simulink model "FOC_PMSM_FVSensorNew"  (R2019b)
settings: Solver=ode45  StartTime=0  StopTime=1  FixedStep=1/fs/4  MaxStep=1/fs/2  RelTol=1e-7  EnableMultiTasking=on
InitFcn:
  | Motor_parameters_Lsrpm7fw
values from neighbouring files (symbols this model uses):
  fs = 20e3    (= 20000)    [Motor_parameters_Lsrpm7fw.m]
  Iphmax = I_rated*sqrt(2)*3    [Motor_parameters_Lsrpm7fw.m]
  J = 1*1e-3    (= 0.001)    [Motor_parameters_Lsrpm7fw.m]
  Ki1 = 2    [Motor_parameters_Lsrpm7fw.m]
  Ki2 = 6000    [Motor_parameters_Lsrpm7fw.m]
  Ki_pll = Bw^2*(1.1-0.334*zeta)^2*1/(2*k1)    (= 1705731.55439)    [Motor_parameters_Lsrpm7fw.m]
  Kp1 = 0.005    [Motor_parameters_Lsrpm7fw.m]
  Kp2 = 6    [Motor_parameters_Lsrpm7fw.m]
  Kp_pll = Bw*(2.2*zeta-0.668*zeta^2)*1/(2*k1)    (= 27920.01984)    [Motor_parameters_Lsrpm7fw.m]
  Ld = 10e-3    (= 0.01)    [Motor_parameters_Lsrpm7fw.m]
  Lndd_ini = Lndmpm    (= 0.412)    [Motor_parameters_Lsrpm7fw.m]
  Lndmpm = 0.412    [Motor_parameters_Lsrpm7fw.m]
  Lq = 12.8e-3    (= 0.0128)    [Motor_parameters_Lsrpm7fw.m]
  Npp = 8/2    (= 4)    [Motor_parameters_Lsrpm7fw.m]
  Omegae_ini = 0    [Motor_parameters_Lsrpm7fw.m]
  Rs = 0.78    [Motor_parameters_Lsrpm7fw.m]
  Tl_const = Trat/nrat^2    (= 1.24081632653e-05)    [Motor_parameters_Lsrpm7fw.m]
  Trat = 38    [Motor_parameters_Lsrpm7fw.m]
  Vm = 70    [Motor_parameters_Lsrpm7fw.m]
  Vph = Vs*sqrt(2)    [Motor_parameters_Lsrpm7fw.m]
undefined symbols (not defined in the file or in its folder): DiscIntNeverNeededParam, plecs, sigbuilder_block
libraries: simulink x1
(part 1 of 2)
settings Model: Creator=klu  LastModifiedBy=Kristina
settings SolverCC: AlgebraicLoopSolver=LineSearch
settings DataIOCC: LimitDataPoints=on  SaveFormat=Array  SignalLoggingSaveFormat=ModelDataLogs  ReturnWorkspaceOutputs=off
settings OptimizationCC: BooleanDataType=off  ExpressionDepthLimit=2147483647  InitFltsAndDblsToZero=on  LifeSpan=inf
settings DebuggingCC: AlgebraicLoopMsg=none  SaveWithParameterizedLinksMsg=none  UnderspecifiedInitializationDetection=Classic  MergeDetectMultiDrivingBlocksExec=none  SignalResolutionControl=TryResolveAllWithWarning  MultiTaskDSMMsg=warning  MultiTaskCondExecSysMsg=none  FcnCallInpInsideContextMsg=warning  StateNameClashWarn=warning  SFUnexpectedBacktrackingDiag=warning  SFNoUnconditionalDefaultTransitionDiag=warning  SFExecutionAtInitializationDiag=none  ArithmeticOperatorsInVariantConditions=warning
settings HardwareCC: ProdBitPerPointer=32  ProdBitPerSizeT=32  ProdBitPerPtrDiffT=32  ProdLargestAtomicFloat=None  ProdIntDivRoundTo=Undefined  ProdEndianess=Unspecified  ProdWordSize=32  ProdHWDeviceType=32-bit Generic
settings ModelReferenceCC: PropagateSignalLabelsOutOfModel=off
settings SFSimCC: SimUseLocalCustomCode=off  CustomCodeUndefinedFunction=UseInterfaceOnly
settings RTWCC: RTWUseLocalCustomCode=off
settings CodeAppCC: StateflowObjectComments=on
settings GRTTargetCC: TargetFcnLib=ansi_tfl_tmw.mat  TargetLangStandard=C89/C90 (ANSI)  GeneratePreprocessorConditionals=Disable all  CombineOutputUpdateFcns=off  GRTInterface=on
settings ConfigComp: CovMetricSettings=dw  CovHtmlReporting=on  CovSaveCumulativeToWorkspaceVar=on  CovSaveSingleToWorkspaceVar=on  CovExternalEMLEnable=off  CovSFcnEnable=off

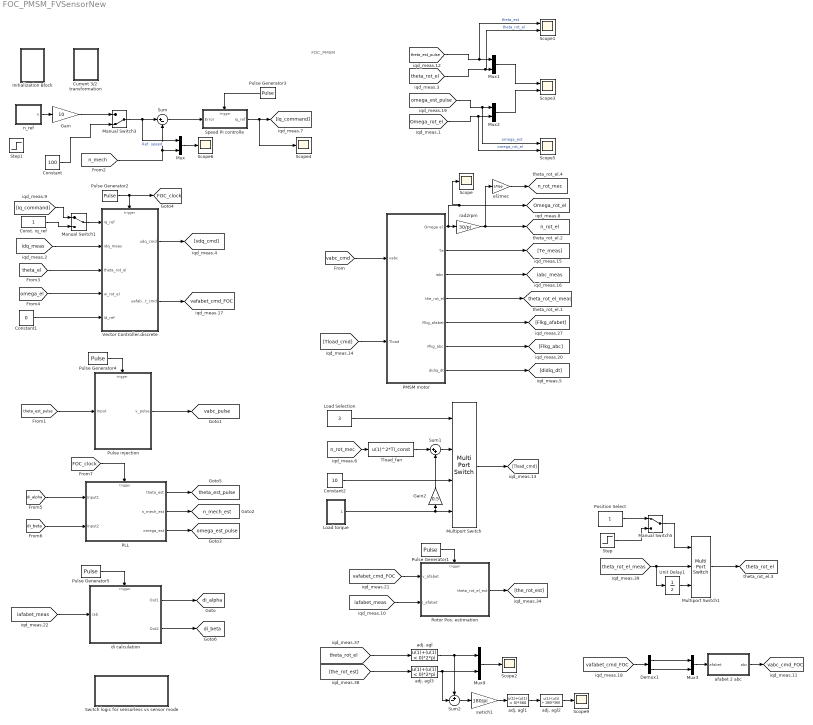
== system FOC_PMSM_FVSensorNew ==
  note: FOC_PMSM
  Const. iq_ref : Constant
  Constant : Constant  Value=100
  Constant1 : Constant  Value=0
  Constant2 : Constant  Value=10
  Current 3/2 transformation : Subsystem
      mask Display:
      | plot([0.1000    0.1357    0.1714    0.2071    0.2429    0.2786    0.3143    0.3500    0.3857    0.4214 0.4571    0.4929    0.5286    0.5643    0.6000]-0.05,0.4+0.6*[0.5000    0.5868    0.6564    0.6950    0.6950    0.6564    0.5868    0.5000    0.4132    0.3436 0.3050    0.3050    0.3436    0.4132    0.5000])
      | 
      | plot([0.1,0.9],[0.1,0.9])
      | 
      | plot([0.5,0.9],0.3*[1 1])
  Demux1 : Demux  Outputs=2
  Gain : Gain  Gain=10
  Gain2 : Gain  Gain=0.5
  Initialization Block : Subsystem  mask{init_in=Motor_parameters_Lsrpm7fw}
      mask prompts: init_in "Enter Initialization Script:"
      mask init:
      | aaa =3;
      mask Callback init_in:
      | init_script=get_param(gcb,'MaskValueString');
      | %eval(init_script);
      | %set_param(gcs,'PreLoadFcn',init_script)
      | set_param(gcs,'InitFcn',init_script)
      | 
      | % Change the parameters here;
      | Ld               = Ld;
      | Lq               = Ld;
  Load Selection : Constant  Value=3
  Load torque : Subsystem
  Manual Switch1 : ManualSwitch
  Manual Switch3 : ManualSwitch  CurrentSetting=0
  Manual Switch5 : ManualSwitch
  Multiport Switch : MultiPortSwitch
  Multiport Switch1 : MultiPortSwitch  Inputs=2
  Mux{,1..3,9} (5 alike) : Mux  Inputs=2
  PLL : Subsystem  TreatAsAtomicUnit=on
  PMSM motor : Subsystem
  Position Select : Constant
  Pulse Generator1 : DiscretePulseGenerator  PulseType=Time based  Period=1/fs  PulseWidth=50  PhaseDelay=1/fs/4*0
  Pulse Generator2 : DiscretePulseGenerator  PulseType=Time based  Period=1/fs  PulseWidth=50
  Pulse Generator3 : DiscretePulseGenerator  PulseType=Time based  Period=1/fs  PulseWidth=50
  Pulse Generator4 : DiscretePulseGenerator  PulseType=Time based  Period=1/fs  PulseWidth=50  PhaseDelay=(1/fs)*0.5
  Pulse Generator5 : DiscretePulseGenerator  PulseType=Time based  Period=1/(fs*2)  PulseWidth=50
  Pulse injection : Subsystem  TreatAsAtomicUnit=on
  Rotor Pos. estimation : Subsystem
  Scope{,2,4,6,9} (5 alike) : Scope
  Scope1 : Scope  NumInputPorts=2
  Scope3 : Scope  NumInputPorts=2
  Scope5 : Scope  NumInputPorts=2
  Speed PI controlle : Subsystem
  Step : Step  Time=0  Before=1  After=2  SampleTime=0
  Step1 : Step  Time=0.2  Before=100  After=100  SampleTime=0
  Sum : Sum  Inputs=|+-
  Sum1 : Sum  Inputs=|++
  Sum2 : Sum  Inputs=+-|
  Switch logic for sensorless vs sensor mode : Subsystem
  Tload_fan : Fcn  Expr=u(1)^2*Tl_const
  Unit Delay1 : UnitDelay  SampleTime=(1/fs)*4  HasFrameUpgradeWarning=on
  Vector Controller.discrete : Subsystem
  adj. agl : Fcn  Expr=u(1)+(u(1) < 0)*2*pi
  adj. agl1 : Fcn  Expr=u(1)+(u(1) < 0)*360
  adj. agl2 : Fcn  Expr=u(1)-(u(1) > 180)*360
  adj. agl3 : Fcn  Expr=u(1)+(u(1) < 0)*2*pi
  afabet 2 abc : Subsystem
  di calculation : Subsystem  TreatAsAtomicUnit=on
  el2mec : Gain  Gain=1/Npp
  n_ref : Subsystem  Tag=STV Subsys  LoadFcn=sigbuilder_block('load');  StartFcn=sigbuilder_block('start');  StopFcn=sigbuilder_block('stop');  ClipboardFcn=sigbuilder_block('clipboard');  mask(Sigbuilder block){tuvar=[0:10]}
      mask help: Sigbuilder GUI
      mask init:
      | if ~strcmp(get_param(bdroot(gcbh),'SimulationStatus'),'stopped') tuvar = sigbuilder_block('maskInit'); end
      settings: CopyFcn=sigbuilder_block('copy');  DeleteFcn=sigbuilder_block('delete');  ModelCloseFcn=sigbuilder_block('modelClose');  PreSaveFcn=sigbuilder_block('preSave');  PauseFcn=sigbuilder_block('pause')  ContinueFcn=sigbuilder_block('continue')  NameChangeFcn=sigbuilder_block('namechange');  OpenFcn=sigbuilder_block('open',[72.75 116.25 550.5 363.75 ]);  CloseFcn=sigbuilder_block('close');
      mask Display: plot(0, 0, 100, 100,[2, 2, 32, 32, 2], [68, 8, 8, 68, 68],[32, 2], [38, 38], [32, 19, 2],[53, 60, 44], [32, 17, 17, 2],[16, 16, 31, 31]);txt = getActiveGroup(gcbh);text(2, 100, txt,'verticalAlignment', 'top');
  rad2rpm : Gain  Gain=30/pi
  swtich1 : Gain  Gain=180/pi
  tag scope: FOC_clock=global, Omega_rot_el=global, di_alpha=global, di_beta=global, iabc_meas=global, n_mech_est=global, n_rot_el=global, n_rot_mec=global, omega_est_pulse=global, theta_est_pulse=global, theta_rot_el=global, theta_rot_el_meas=global, vabc_cmd_FOC=global, vabc_pulse=global, vafabet_cmd_FOC=global
  wires:
  Manual Switch1/1 -> Vector Controller.discrete/1(iq_ref)
  Const. iq_ref/1 -> Manual Switch1/2
  Sum/1 -> Speed PI controlle/1(Error)
  [idq_meas] -> Vector Controller.discrete/2(idq_meas)
  Vector Controller.discrete/1(udq_cmd) -> [vdq_cmd]
  Vector Controller.discrete/2(uafabet_cmd) -> [vafabet_cmd_FOC]
  Constant2/1 -> Multiport Switch/3
  Load torque/1(T_load) -> Multiport Switch/4, Gain2/1
  Multiport Switch/1 -> [Tload_cmd]
  [n_rot_mec] -> Tload_fan/1
  Load Selection/1 -> Multiport Switch/1
  [theta_rot_el_meas] -> Unit Delay1/1, Multiport Switch1/2
  Multiport Switch1/1 -> [theta_rot_el]
  Position Select/1 -> Manual Switch5/1
  Step/1 -> Manual Switch5/2
  Manual Switch5/1 -> Multiport Switch1/1
  n_ref/1(n) -> Gain/1
  Gain/1 -> Manual Switch3/1
  Sum1/1 -> Multiport Switch/2
  Tload_fan/1 -> Sum1/1
  [theta_el] -> Vector Controller.discrete/3(theta_rot_el)
  Constant1/1 -> Vector Controller.discrete/5(Id_ref)
  Gain2/1 -> Sum1/2
  Unit Delay1/1 -> Multiport Switch1/3
  [omega_el] -> Vector Controller.discrete/4(w_rot_el)
  PMSM motor/2(Te) -> [Te_meas]
  PMSM motor/1(Omega el.) -> Scope/1, [Omega_rot_el], rad2rpm/1
  rad2rpm/1 -> [n_rot_el], el2mec/1
  PMSM motor/5(Flkg_afabet) -> [Flkg_afabet]
  PMSM motor/6(Flkg_abc) -> [Flkg_abc]
  [Tload_cmd] -> PMSM motor/2(Tload)
  PMSM motor/3(iabc) -> [iabc_meas]
  PMSM motor/7(didiq_dt) -> [didiq_dt]
  Demux1/2 -> Mux3/2
  Demux1/1 -> Mux3/1
  [vafabet_cmd_FOC] -> Demux1/1
  afabet 2 abc/1(abc) -> [vabc_cmd_FOC]
  Mux3/1 -> afabet 2 abc/1(afabet)
  Speed PI controlle/1(iq_ref) -> Scope4/1, [Iq_command]
  [Iq_command] -> Manual Switch1/1
  adj. agl1/1 -> adj. agl2/1
  [the_rot_est] -> adj. agl3/1
  adj. agl2/1 -> Scope9/1
  [iafabet_meas] -> Rotor Pos. estimation/2(i_afabet)
  swtich1/1 -> adj. agl1/1
  Sum2/1 -> swtich1/1
  [vafabet_cmd_FOC] -> Rotor Pos. estimation/1(v_afabet)
  Rotor Pos. estimation/1(theta_rot_el_est) -> [the_rot_est]
  adj. agl/1 -> Mux9/1, Sum2/1
  [theta_rot_el] -> adj. agl/1
  Pulse Generator1/1 -> Rotor Pos. estimation/Trigger
  adj. agl3/1 -> Mux9/2, Sum2/2
  el2mec/1 -> [n_rot_mec]
  Pulse Generator3/1 -> Speed PI controlle/Trigger
  Mux9/1 -> Scope2/1
  Pulse Generator4/1 -> Pulse injection/Trigger
  Pulse Generator2/1 -> [FOC_clock], Vector Controller.discrete/Trigger
  [iafabet_meas] -> di calculation/1(iab)
  Pulse injection/1(v_pulse) -> [vabc_pulse]
  Manual Switch3/1 -> Mux/1, Sum/1  "Ref. speed"
  Mux/1 -> Scope6/1
  [n_mech] -> Mux/2, Sum/2
  [vabc_cmd] -> PMSM motor/1(vabc)
  Pulse Generator5/1 -> di calculation/Trigger
  PMSM motor/4(the_rot_el) -> [theta_rot_el_meas]
  PLL/1(theta_est) -> [theta_est_pulse]
  PLL/2(n_mech_est) -> [n_mech_est]
  PLL/3(omega_est) -> [omega_est_pulse]
  [theta_est_pulse] -> Pulse injection/1(Input)
  di calculation/1(Out1) -> [di_alpha]
  di calculation/2(Out2) -> [di_beta]
  [di_alpha] -> PLL/1(Input1)
  [di_beta] -> PLL/2(Input2)
  [FOC_clock] -> PLL/Trigger
  [theta_est_pulse] -> Scope1/1, Mux1/1  "theta_est"
  [theta_rot_el] -> Scope1/2, Mux1/2  "theta_rot_el"
  [omega_est_pulse] -> Scope5/1, Mux2/1  "omega_est"
  [Omega_rot_el] -> Scope5/2, Mux2/2  "omega_rot_el"
  Mux1/1 -> Scope3/1
  Mux2/1 -> Scope3/2
  Constant/1 -> Manual Switch3/2

== system FOC_PMSM_FVSensorNew/Current 3//2 transformation ==
  Delay : Delay  DelayLength=1
  Detect peak : Subsystem
  Display : Display
  Display1 : Display
  Manual Switch7 : ManualSwitch  CurrentSetting=0
  Scope14 : Scope
  Scope6 : Scope
  abc 2 dq : Subsystem
  dq 2 afa beta : Subsystem
  tag scope: iafabet_meas=global, idq_meas=global
  wires:
  abc 2 dq/1(dq) -> [idq_meas], Scope6/1, dq 2 afa beta/1(dq)
  dq 2 afa beta/1(afa beta) -> [iafabet_meas], Scope14/1
  Manual Switch7/1 -> abc 2 dq/1(abc), Detect peak/1(iabc)
  Detect peak/1(Peak) -> Display/1
  [iabc_meas] -> Manual Switch7/1, Manual Switch7/2
  [theta_el] -> Delay/1, Display1/1
  Delay/1 -> abc 2 dq/2(theta), dq 2 afa beta/2(theta)

== system FOC_PMSM_FVSensorNew/Initialization Block ==

== system FOC_PMSM_FVSensorNew/Load torque ==
  Add : Sum  Inputs=+++
  Scope2 : Scope
  Step Load torque 1 : Step  Time=2  After=Trat  SampleTime=0
  Step Load torque2 : Step  Time=4  After=-Trat/2  SampleTime=0
  Tload : Constant  Value=0
  T_load : Outport  VectorParamsAs1DForOutWhenUnconnected=off
  wires:
  Tload/1 -> Add/1
  Step Load torque 1/1 -> Add/2
  Step Load torque2/1 -> Add/3
  Add/1 -> T_load/1, Scope2/1

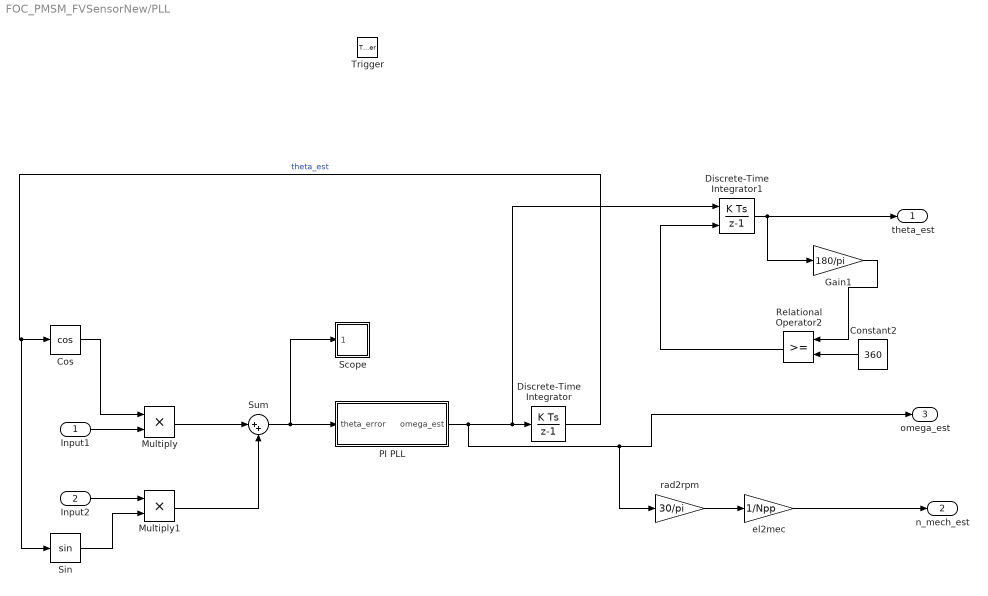
== system FOC_PMSM_FVSensorNew/PLL ==
  Input1 : Inport
  Input2 : Inport  Port=2
  Trigger : TriggerPort  VariantControl=Variant
  Constant2 : Constant  Value=360
  Cos : Trigonometry  Operator=cos
  Discrete-Time Integrator : DiscreteIntegrator  SampleTime=-1  ICPrevOutput=DiscIntNeverNeededParam  ICPrevScaledInput=DiscIntNeverNeededParam
  Discrete-Time Integrator1 : DiscreteIntegrator  ExternalReset=rising  SampleTime=-1  ICPrevOutput=DiscIntNeverNeededParam  ICPrevScaledInput=DiscIntNeverNeededParam
  Gain1 : Gain  Gain=180/pi
  Multiply : Product
  Multiply1 : Product
  PI PLL : Subsystem
  Relational Operator2 : RelationalOperator  OutDataTypeStr=boolean  RndMeth=Nearest
  Scope : Subsystem  LoadFcn=plecs('sl', 300);  InitFcn=plecs('sl', 314);  StartFcn=plecs('sl', 308);  StopFcn=plecs('sl', 309);  mask{Settings=<binary blob, 232 chars, not shown>}
      mask init:
      | plecs('sl', 315);
      settings: CopyFcn=plecs('sl', 303);  DeleteFcn=plecs('sl', 305);  UndoDeleteFcn=plecs('sl', 306);  PreSaveFcn=plecs('sl', 311);  NameChangeFcn=plecs('sl', 310);  DestroyFcn=plecs('sl', 307);  OpenFcn=plecs('sl', 302);  ErrorFcn=plerrorfcn
      mask Display: plot([0.1 0.9 0.9 0.1 0.1], [0.9 0.9 0.5 0.5 0.9])
  Sin : Trigonometry
  Sum : Sum  Inputs=|++
  el2mec : Gain  Gain=1/Npp
  rad2rpm : Gain  Gain=30/pi
  theta_est : Outport  VectorParamsAs1DForOutWhenUnconnected=off
  n_mech_est : Outport  Port=2  VectorParamsAs1DForOutWhenUnconnected=off
  omega_est : Outport  Port=3  VectorParamsAs1DForOutWhenUnconnected=off
  wires:
  el2mec/1 -> n_mech_est/1
  Sum/1 -> Scope/1(1), PI PLL/1(theta_error)
  Multiply/1 -> Sum/1
  Relational Operator2/1 -> Discrete-Time Integrator1/2
  Input2/1 -> Multiply1/1
  Gain1/1 -> Relational Operator2/1
  Discrete-Time Integrator1/1 -> Gain1/1, theta_est/1
  Cos/1 -> Multiply/1
  Sin/1 -> Multiply1/2
  Input1/1 -> Multiply/2
  rad2rpm/1 -> el2mec/1
  Discrete-Time Integrator/1 -> Sin/1, Cos/1  "theta_est"
  PI PLL/1(omega_est) -> rad2rpm/1, omega_est/1, Discrete-Time Integrator1/1, Discrete-Time Integrator/1
  Constant2/1 -> Relational Operator2/2
  Multiply1/1 -> Sum/2

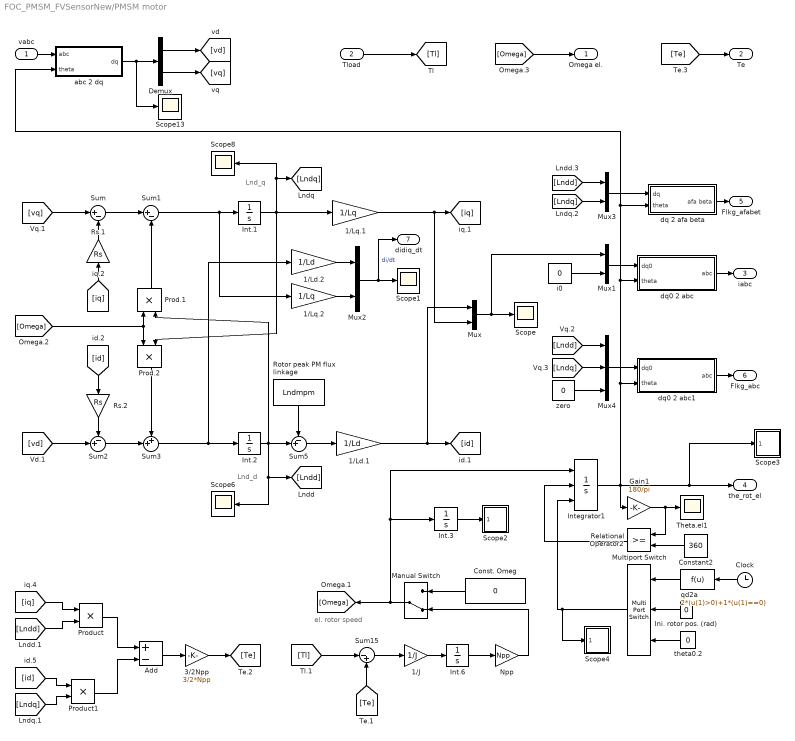
== system FOC_PMSM_FVSensorNew/PMSM motor ==
  note: Lnd_d
  note: Lnd_q
  note: el. rotor speed
  vabc : Inport
  Tload : Inport  Port=2
  1/J : Gain  Gain=1/J
  1/Ld.1 : Gain  Gain=1/Ld
  1/Ld.2 : Gain  Gain=1/Ld
  1/Lq.1 : Gain  Gain=1/Lq
  1/Lq.2 : Gain  Gain=1/Lq
  3/2Npp : Gain  Gain=3/2*Npp
  Add : Sum  Inputs=+-
  Clock : Clock
  Const. Omeg : Constant  Value=0
  Constant2 : Constant  Value=360
  Demux : Demux  Outputs=2
  Gain1 : Gain  Gain=180/pi
  Ini. rotor pos. (rad) : Constant  Value=0
  Int.1 : Integrator
  Int.2 : Integrator  InitialCondition=Lndd_ini
  Int.3 : Integrator  InitialCondition=Omegae_ini/Npp
  Int.6 : Integrator  InitialCondition=Omegae_ini/Npp
  Integrator1 : Integrator  ExternalReset=rising  InitialConditionSource=external  InitialCondition=pi/3
  Manual Switch : ManualSwitch  CurrentSetting=0
  Multiport Switch : MultiPortSwitch  Inputs=2
  Mux{,1..3} (4 alike) : Mux  Inputs=2
  Mux4 : Mux  Inputs=3
  Npp : Gain  Gain=Npp
  Prod.1 : Product  RndMeth=Zero
  Prod.2 : Product  RndMeth=Zero
  Product : Product  RndMeth=Zero
  Product1 : Product  RndMeth=Zero
  Relational Operator2 : RelationalOperator  OutDataTypeStr=boolean  RndMeth=Nearest
  Rotor peak PM flux linkage : Constant  Value=Lndmpm
  Rs.1 : Gain  Gain=Rs
  Rs.2 : Gain  Gain=Rs
  Scope{,1,6,8,13} (5 alike) : Scope
  Scope2 : Subsystem  LoadFcn=plecs('sl', 300);  InitFcn=plecs('sl', 314);  StartFcn=plecs('sl', 308);  StopFcn=plecs('sl', 309);  mask{Settings=<binary blob, 1052 chars, not shown>}
      mask init:
      | plecs('sl', 315);
      settings: CopyFcn=plecs('sl', 303);  DeleteFcn=plecs('sl', 305);  UndoDeleteFcn=plecs('sl', 306);  PreSaveFcn=plecs('sl', 311);  NameChangeFcn=plecs('sl', 310);  DestroyFcn=plecs('sl', 307);  OpenFcn=plecs('sl', 302);  ErrorFcn=plerrorfcn
      mask Display: plot([0.1 0.9 0.9 0.1 0.1], [0.9 0.9 0.5 0.5 0.9])
  Scope3 : Subsystem  LoadFcn=plecs('sl', 300);  InitFcn=plecs('sl', 314);  StartFcn=plecs('sl', 308);  StopFcn=plecs('sl', 309);  mask{Settings=<binary blob, 1052 chars, not shown>}
      mask init:
      | plecs('sl', 315);
      settings: CopyFcn=plecs('sl', 303);  DeleteFcn=plecs('sl', 305);  UndoDeleteFcn=plecs('sl', 306);  PreSaveFcn=plecs('sl', 311);  NameChangeFcn=plecs('sl', 310);  DestroyFcn=plecs('sl', 307);  OpenFcn=plecs('sl', 302);  ErrorFcn=plerrorfcn
      mask Display: plot([0.1 0.9 0.9 0.1 0.1], [0.9 0.9 0.5 0.5 0.9])
  Scope4 : Subsystem  LoadFcn=plecs('sl', 300);  InitFcn=plecs('sl', 314);  StartFcn=plecs('sl', 308);  StopFcn=plecs('sl', 309);  mask{Settings=<binary blob, 1052 chars, not shown>}
      mask init:
      | plecs('sl', 315);
      settings: CopyFcn=plecs('sl', 303);  DeleteFcn=plecs('sl', 305);  UndoDeleteFcn=plecs('sl', 306);  PreSaveFcn=plecs('sl', 311);  NameChangeFcn=plecs('sl', 310);  DestroyFcn=plecs('sl', 307);  OpenFcn=plecs('sl', 302);  ErrorFcn=plerrorfcn
      mask Display: plot([0.1 0.9 0.9 0.1 0.1], [0.9 0.9 0.5 0.5 0.9])
  Sum : Sum  Inputs=|+-
  Sum1 : Sum  Inputs=|+-
  Sum15 : Sum  Inputs=|-+
  Sum2 : Sum  Inputs=-+|
  Sum3 : Sum  Inputs=++|
  Sum5 : Sum  Inputs=-+|
  Theta.el1 : Scope
  abc 2 dq : Subsystem
  dq 2 afa beta : Subsystem
  dq0 2 abc : Subsystem
  dq0 2 abc1 : Subsystem
  i0 : Constant  Value=0
  qd2a : Fcn  Expr=2*(u(1)>0)+1*(u(1)==0)
  theta0.2 : Constant  Value=0
  zero : Constant  Value=0
  Omega el. : Outport  VectorParamsAs1DForOutWhenUnconnected=off
  Te : Outport  Port=2  VectorParamsAs1DForOutWhenUnconnected=off
  iabc : Outport  Port=3  VectorParamsAs1DForOutWhenUnconnected=off
  the_rot_el : Outport  Port=4  VectorParamsAs1DForOutWhenUnconnected=off
  Flkg_afabet : Outport  Port=5  VectorParamsAs1DForOutWhenUnconnected=off
  Flkg_abc : Outport  Port=6  VectorParamsAs1DForOutWhenUnconnected=off
  didiq_dt : Outport  Port=7  VectorParamsAs1DForOutWhenUnconnected=off
  wires:
  3/2Npp/1 -> [Te]
  Add/1 -> 3/2Npp/1
  Sum5/1 -> 1/Ld.1/1
  Rotor peak PM flux linkage/1 -> Sum5/1
  [Omega] -> Omega el./1
  [Te] -> Te/1
  Product1/1 -> Add/2
  Product/1 -> Add/1
  [Lndq] -> Product1/2
  [id] -> Product1/1
  [Te] -> Sum15/2
  Int.6/1 -> Npp/1
  1/J/1 -> Int.6/1
  Sum15/1 -> 1/J/1
  [Tl] -> Sum15/1
  Mux/1 -> Scope/1, Mux1/1
  [Omega] -> Prod.2/1, Prod.1/1
  Sum3/1 -> Int.2/1, 1/Ld.2/1
  Prod.2/1 -> Sum3/1
  Sum2/1 -> Sum3/2
  [id] -> Rs.2/1
  Rs.2/1 -> Sum2/1
  [vd] -> Sum2/2
  1/Ld.1/1 -> [id], Mux/1
  Int.2/1 -> [Lndd], Scope6/1, Sum5/2, Prod.1/2
  [iq] -> Rs.1/1
  1/Lq.1/1 -> [iq], Mux/2
  Prod.1/1 -> Sum1/2
  Sum1/1 -> Int.1/1, 1/Lq.2/1
  Int.1/1 -> 1/Lq.1/1, Prod.2/2, Scope8/1, [Lndq]
  Sum/1 -> Sum1/1
  Rs.1/1 -> Sum/2
  [vq] -> Sum/1
  Tload/1 -> [Tl]
  Demux/2 -> [vq]
  Demux/1 -> [vd]
  i0/1 -> Mux1/2
  Mux1/1 -> dq0 2 abc/1(dq0)
  dq0 2 abc/1(abc) -> iabc/1
  vabc/1 -> abc 2 dq/1(abc)
  abc 2 dq/1(dq) -> Demux/1, Scope13/1
  Integrator1/1 -> Scope3/1(1), the_rot_el/1, dq0 2 abc/2(theta), dq 2 afa beta/2(theta), abc 2 dq/2(theta), dq0 2 abc1/2(theta), Gain1/1
  1/Ld.2/1 -> Mux2/1
  1/Lq.2/1 -> Mux2/2
  Mux2/1 -> didiq_dt/1, Scope1/1  "di/dt"
  Mux3/1 -> dq 2 afa beta/1(dq)
  [Lndd] -> Mux3/1
  [Lndq] -> Mux3/2
  dq 2 afa beta/1(afa beta) -> Flkg_afabet/1
  [Lndd] -> Mux4/1
  [Lndq] -> Mux4/2
  Mux4/1 -> dq0 2 abc1/1(dq0)
  dq0 2 abc1/1(abc) -> Flkg_abc/1
  zero/1 -> Mux4/3
  Gain1/1 -> Theta.el1/1, Relational Operator2/1
  Constant2/1 -> Relational Operator2/2
  [iq] -> Product/1
  [Lndd] -> Product/2
  Relational Operator2/1 -> Integrator1/2
  Ini. rotor pos. (rad)/1 -> Multiport Switch/2
  theta0.2/1 -> Multiport Switch/3
  qd2a/1 -> Multiport Switch/1
  Clock/1 -> qd2a/1
  Multiport Switch/1 -> Scope4/1(1), Integrator1/3
  Const. Omeg/1 -> Manual Switch/1
  Npp/1 -> Manual Switch/2
  Manual Switch/1 -> Int.3/1, Integrator1/1, [Omega]
  Int.3/1 -> Scope2/1(1)

== system FOC_PMSM_FVSensorNew/Pulse injection ==
  Input : Inport
  Trigger : TriggerPort  VariantControl=Variant
  Constant : Constant  Value=0
  Constant1 : Constant  Value=Vm
  Mux : Mux  Inputs=2
  afabet 2 abc : Subsystem
  dq 2 afa beta : Subsystem
  v_pulse : Outport  VectorParamsAs1DForOutWhenUnconnected=off
  wires:
  Constant/1 -> Mux/1
  Constant1/1 -> Mux/2
  Mux/1 -> dq 2 afa beta/1(dq)
  dq 2 afa beta/1(afa beta) -> afabet 2 abc/1(afabet)
  afabet 2 abc/1(abc) -> v_pulse/1
  Input/1 -> dq 2 afa beta/2(theta)

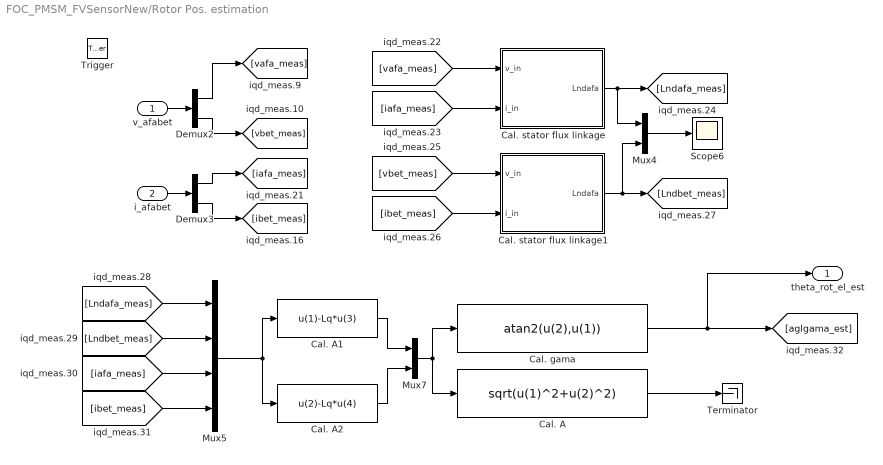
== system FOC_PMSM_FVSensorNew/Rotor Pos. estimation ==
  v_afabet : Inport  LatchByDelayingOutsideSignal=on
  i_afabet : Inport  Port=2  LatchByDelayingOutsideSignal=on
  Trigger : TriggerPort  VariantControl=(inherit)
  Cal. A : Fcn  Expr=sqrt(u(1)^2+u(2)^2)
  Cal. A1 : Fcn  Expr=u(1)-Lq*u(3)
  Cal. A2 : Fcn  Expr=u(2)-Lq*u(4)
  Cal. gama : Fcn  Expr=atan2(u(2),u(1))
  Cal. stator flux linkage : Subsystem
  Cal. stator flux linkage1 : Subsystem
  Demux2 : Demux  Outputs=2
  Demux3 : Demux  Outputs=2
  Mux4 : Mux  Inputs=2
  Mux5 : Mux
  Mux7 : Mux  Inputs=2
  Scope6 : Scope
  Terminator : Terminator
  theta_rot_el_est : Outport  VectorParamsAs1DForOutWhenUnconnected=off
  wires:
  Demux2/1 -> [vafa_meas]
  Demux2/2 -> [vbet_meas]
  Demux3/1 -> [iafa_meas]
  Demux3/2 -> [ibet_meas]
  [vafa_meas] -> Cal. stator flux linkage/1(v_in)
  [iafa_meas] -> Cal. stator flux linkage/2(i_in)
  Cal. stator flux linkage/1(Lndafa) -> [Lndafa_meas], Mux4/1
  [vbet_meas] -> Cal. stator flux linkage1/1(v_in)
  [ibet_meas] -> Cal. stator flux linkage1/2(i_in)
  Cal. stator flux linkage1/1(Lndafa) -> [Lndbet_meas], Mux4/2
  Mux4/1 -> Scope6/1
  [Lndafa_meas] -> Mux5/1
  [Lndbet_meas] -> Mux5/2
  [iafa_meas] -> Mux5/3
  [ibet_meas] -> Mux5/4
  Mux5/1 -> Cal. A1/1, Cal. A2/1
  Cal. A1/1 -> Mux7/1
  Cal. A2/1 -> Mux7/2
  Mux7/1 -> Cal. gama/1, Cal. A/1
  Cal. A/1 -> Terminator/1
  v_afabet/1 -> Demux2/1
  i_afabet/1 -> Demux3/1
  Cal. gama/1 -> theta_rot_el_est/1, [aglgama_est]

== system FOC_PMSM_FVSensorNew/Speed PI controlle ==
  Error : Inport
  Trigger : TriggerPort  VariantControl=(inherit)
  Discrete-Time Integrator : DiscreteIntegrator  SampleTime=-1  ICPrevOutput=DiscIntNeverNeededParam  ICPrevScaledInput=DiscIntNeverNeededParam
  Kp : Gain  Gain=Kp1
  Sum1 : Sum  Inputs=|++
  ki : Gain  Gain=Ki1
  iq_ref : Outport  VectorParamsAs1DForOutWhenUnconnected=off
  wires:
  Kp/1 -> Sum1/1
  ki/1 -> Discrete-Time Integrator/1
  Discrete-Time Integrator/1 -> Sum1/2
  Sum1/1 -> iq_ref/1
  Error/1 -> Kp/1, ki/1

== system FOC_PMSM_FVSensorNew/Switch logic for sensorless vs sensor mode ==
  Scope : Scope
  Switch : Switch  Criteria=u2 > Threshold  Threshold=0.5
  Terminator1 : Terminator
  Terminator2 : Terminator
  Terminator3 : Terminator
  tag scope: n_mech=global, omega_el=global, theta_el=global, vabc_cmd=global
  wires:
  [n_rot_mec] -> [n_mech]
  [theta_est_pulse] -> [theta_el]
  [vabc_cmd_FOC] -> Switch/1
  [vabc_pulse] -> Switch/3
  [FOC_clock] -> Switch/2
  Switch/1 -> Scope/1, [vabc_cmd]
  [omega_est_pulse] -> [omega_el]
  [theta_rot_el] -> Terminator1/1
  [n_mech_est] -> Terminator2/1
  [Omega_rot_el] -> Terminator3/1

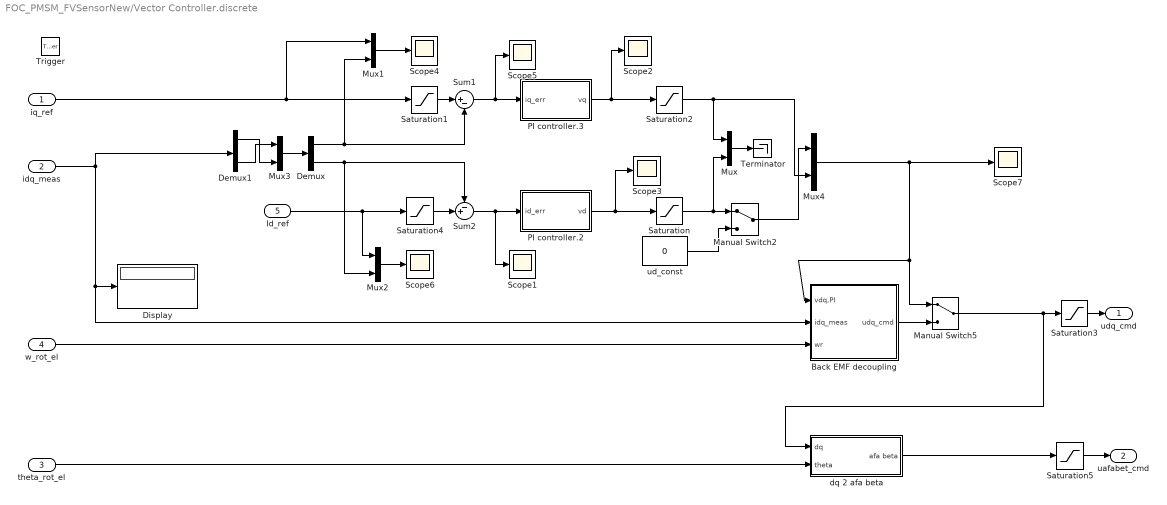
== system FOC_PMSM_FVSensorNew/Vector Controller.discrete ==
  iq_ref : Inport
  idq_meas : Inport  Port=2
  theta_rot_el : Inport  Port=3
  w_rot_el : Inport  Port=4
  Id_ref : Inport  Port=5
  Trigger : TriggerPort  VariantControl=(inherit)
  Back EMF decoupling : Subsystem
  Demux : Demux  Outputs=2
  Demux1 : Demux  Outputs=2
  Display : Display
  Manual Switch2 : ManualSwitch
  Manual Switch5 : ManualSwitch
  Mux{,1..4} (5 alike) : Mux  Inputs=2
  PI controller.2 : Subsystem
  PI controller.3 : Subsystem
  Saturation{,2..3,5} (4 alike) : Saturate  UpperLimit=Vph  LowerLimit=-Vph
  Saturation1 : Saturate  UpperLimit=Iphmax  LowerLimit=-Iphmax
  Saturation4 : Saturate  UpperLimit=Iphmax  LowerLimit=-Iphmax
  Scope{1..7} (7 alike) : Scope
  Sum1 : Sum  Inputs=|+-
  Sum2 : Sum  Inputs=-+|
  Terminator : Terminator
  dq 2 afa beta : Subsystem
  ud_const : Constant  Value=0
  udq_cmd : Outport  VectorParamsAs1DForOutWhenUnconnected=off
  uafabet_cmd : Outport  Port=2  VectorParamsAs1DForOutWhenUnconnected=off
  wires:
  Saturation4/1 -> Sum2/2
  Saturation/1 -> Mux/2, Manual Switch2/1
  Mux/1 -> Terminator/1
  PI controller.3/1(vq) -> Scope2/1, Saturation2/1
  Demux/1 -> Sum1/2, Mux1/2
  PI controller.2/1(vd) -> Saturation/1, Scope3/1
  Demux/2 -> Sum2/1, Mux2/2
  Sum1/1 -> Scope5/1, PI controller.3/1(iq_err)
  iq_ref/1 -> Mux1/1, Saturation1/1
  Sum2/1 -> Scope1/1, PI controller.2/1(id_err)
  Id_ref/1 -> Saturation4/1, Mux2/1
  Mux1/1 -> Scope4/1
  Saturation1/1 -> Sum1/1
  Mux2/1 -> Scope6/1
  Saturation2/1 -> Mux/1, Mux4/2
  Manual Switch2/1 -> Mux4/1
  ud_const/1 -> Manual Switch2/2
  Demux1/2 -> Mux3/1
  Demux1/1 -> Mux3/2
  theta_rot_el/1 -> dq 2 afa beta/2(theta)
  dq 2 afa beta/1(afa beta) -> Saturation5/1
  w_rot_el/1 -> Back EMF decoupling/3(wr)
  Back EMF decoupling/1(udq_cmd) -> Manual Switch5/2
  Mux4/1 -> Scope7/1, Manual Switch5/1, Back EMF decoupling/1(vdq,PI)
  Manual Switch5/1 -> dq 2 afa beta/1(dq), Saturation3/1
  Mux3/1 -> Demux/1
  idq_meas/1 -> Demux1/1, Display/1, Back EMF decoupling/2(idq_meas)
  Saturation3/1 -> udq_cmd/1
  Saturation5/1 -> uafabet_cmd/1

== system FOC_PMSM_FVSensorNew/afabet 2 abc ==
  afabet : Inport
  Constant : Constant  Value=0
  Mux1 : Mux  Inputs=2
  Mux2 : Mux  Inputs=3
  qd2a : Fcn  Expr=u(1)+u(3)
  qd2b : Fcn  Expr=u(1)*cos(2/3*pi)+u(2)*sin(2/3*pi)+u(3)
  qd2c : Fcn  Expr=u(1)*cos(2/3*pi)-u(2)*sin(2/3*pi)+u(3)
  abc : Outport  VectorParamsAs1DForOutWhenUnconnected=off
  wires:
  Constant/1 -> Mux1/2
  qd2c/1 -> Mux2/3
  afabet/1 -> Mux1/1
  Mux1/1 -> qd2c/1, qd2b/1, qd2a/1
  qd2a/1 -> Mux2/1
  qd2b/1 -> Mux2/2
  Mux2/1 -> abc/1

== system FOC_PMSM_FVSensorNew/di calculation ==
  iab : Inport
  Trigger : TriggerPort  VariantControl=Variant
  Delay2 : Delay  DelayLength=1
  Delay3 : Delay  DelayLength=1
  Demux : Demux  Outputs=2
  Scope : Scope  NumInputPorts=2
  Subtract : Sum  Inputs=+-
  Subtract1 : Sum  Inputs=+-
  Out1 : Outport  VectorParamsAs1DForOutWhenUnconnected=off
  Out2 : Outport  Port=2  VectorParamsAs1DForOutWhenUnconnected=off
  wires:
  Demux/1 -> Scope/1, Subtract/1, Delay2/1  "ia0"
  Demux/2 -> Delay3/1, Subtract1/1  "ib0"
  iab/1 -> Demux/1
  Delay2/1 -> Scope/2, Subtract/2  "ia1"
  Delay3/1 -> Subtract1/2  "ib1"
  Subtract/1 -> Out1/1
  Subtract1/1 -> Out2/1

== system FOC_PMSM_FVSensorNew/n_ref ==
  Demux : Demux  Tag=STV Demux  Outputs=1
  FromWs : FromWorkspace  Tag=STV FromWs  VariableName=tuvar  SampleTime=0
      SigBuilderData=|
      | common.afterFinalStr = 'Extrapolate'
      | common.sampleTime = 0
      | dataSet.timeRange = [0 10]
      | dataSet.name = 'Group 1'
      | sbobj.Groups.Name = 'Group 1'
      | sbobj.Groups.Signals.Name = 'n'
      | sbobj.Groups.Signals.XData = [0 1 1 6 6 7 10]
      | sbobj.Groups.Signals.YData = [0 0 0.995 0.995 1 0.39 0.1]
  n : Outport  Tag=STV Outport  VectorParamsAs1DForOutWhenUnconnected=off
  wires:
  Demux/1 -> n/1
  FromWs/1 -> Demux/1

== system FOC_PMSM_FVSensorNew/Current 3//2 transformation/Detect peak ==
  iabc : Inport
  Clock : Clock
  Compare To Constant : simulink/Logic and Bit Operations/Compare To Constant  relop=>=  const=2  OutDataTypeStr=uint8  ZeroCross=off
  Demux1 : Demux  Outputs=3
  MinMax : MinMax  Function=max  Inputs=2
  Product : Product  RndMeth=Zero
  Terminator : Terminator
  Terminator1 : Terminator
  Unit Delay : UnitDelay  SampleTime=1/5e3  HasFrameUpgradeWarning=on
  Peak : Outport  VectorParamsAs1DForOutWhenUnconnected=off
  wires:
  iabc/1 -> Demux1/1
  Demux1/3 -> Terminator/1
  Demux1/2 -> Terminator1/1
  Clock/1 -> Compare To Constant/1
  Compare To Constant/1 -> Product/1
  Demux1/1 -> Product/2
  MinMax/1 -> Peak/1, Unit Delay/1
  Product/1 -> MinMax/1
  Unit Delay/1 -> MinMax/2

== system FOC_PMSM_FVSensorNew/Current 3//2 transformation/abc 2 dq ==
  abc : Inport
  theta : Inport  Port=2
  Mux1 : Mux  Inputs=2
  Mux2 : Mux  Inputs=2
  abc2d : Fcn  Expr=2/3*(u(1)*cos(u(4))+u(2)*cos(u(4)-2*pi/3)+u(3)*cos(u(4)-4*pi/3))
  abc2q : Fcn  Expr=-1*2/3*(u(1)*sin(u(4))+u(2)*sin(u(4)-2*pi/3)+u(3)*sin(u(4)-4*pi/3))
  dq : Outport  VectorParamsAs1DForOutWhenUnconnected=off
  wires:
  Mux2/1 -> dq/1
  abc2q/1 -> Mux2/2
  abc2d/1 -> Mux2/1
  Mux1/1 -> abc2q/1, abc2d/1
  theta/1 -> Mux1/2
  abc/1 -> Mux1/1

== system FOC_PMSM_FVSensorNew/Current 3//2 transformation/dq 2 afa beta ==
  dq : Inport
  theta : Inport  Port=2
  Mux1 : Mux  Inputs=2
  Mux2 : Mux  Inputs=2
  dq2afa : Fcn  Expr=u(1)*cos(u(3))-u(2)*sin(u(3))
  dq2beta : Fcn  Expr=u(1)*sin(u(3))+u(2)*cos(u(3))
  afa beta : Outport  VectorParamsAs1DForOutWhenUnconnected=off
  wires:
  dq/1 -> Mux1/1
  theta/1 -> Mux1/2
  Mux1/1 -> dq2beta/1, dq2afa/1
  dq2afa/1 -> Mux2/1
  dq2beta/1 -> Mux2/2
  Mux2/1 -> afa beta/1

== system FOC_PMSM_FVSensorNew/PLL/PI PLL ==
  theta_error : Inport
  Discrete-Time Integrator : DiscreteIntegrator  SampleTime=-1  ICPrevOutput=DiscIntNeverNeededParam  ICPrevScaledInput=DiscIntNeverNeededParam
  Kp : Gain  Gain=Kp_pll
  Sum1 : Sum  Inputs=|++
  ki : Gain  Gain=Ki_pll
  omega_est : Outport  VectorParamsAs1DForOutWhenUnconnected=off
  wires:
  Sum1/1 -> omega_est/1
  Discrete-Time Integrator/1 -> Sum1/2
  ki/1 -> Discrete-Time Integrator/1
  Kp/1 -> Sum1/1
  theta_error/1 -> ki/1, Kp/1

== system FOC_PMSM_FVSensorNew/PLL/Scope ==
  1 : Inport
  " InputMux " : Subsystem
      mask Display: disp('Mux')
  " S-Function " : S-Function  FunctionName=plecs  SFunctionDeploymentMode=off  EnableBusSupport=off
  wires:
  1/1 -> " InputMux "/1(In1)
  " InputMux "/1(Out) -> " S-Function "/1

== system FOC_PMSM_FVSensorNew/PMSM motor/Scope2 ==
  1 : Inport
  " InputMux " : Subsystem
      mask Display: disp('Mux')
  " S-Function " : S-Function  FunctionName=plecs  SFunctionDeploymentMode=off  EnableBusSupport=off
  wires:
  1/1 -> " InputMux "/1(In1)
  " InputMux "/1(Out) -> " S-Function "/1

== system FOC_PMSM_FVSensorNew/PMSM motor/Scope3 ==
  1 : Inport
  " InputMux " : Subsystem
      mask Display: disp('Mux')
  " S-Function " : S-Function  FunctionName=plecs  SFunctionDeploymentMode=off  EnableBusSupport=off
  wires:
  " InputMux "/1(Out) -> " S-Function "/1
  1/1 -> " InputMux "/1(In1)

== system FOC_PMSM_FVSensorNew/PMSM motor/Scope4 ==
  1 : Inport
  " InputMux " : Subsystem
      mask Display: disp('Mux')
  " S-Function " : S-Function  FunctionName=plecs  SFunctionDeploymentMode=off  EnableBusSupport=off
  wires:
  1/1 -> " InputMux "/1(In1)
  " InputMux "/1(Out) -> " S-Function "/1

== system FOC_PMSM_FVSensorNew/PMSM motor/abc 2 dq ==
  abc : Inport
  theta : Inport  Port=2
  Mux1 : Mux  Inputs=2
  Mux2 : Mux  Inputs=2
  abc2d : Fcn  Expr=-1*2/3*(u(1)*sin(u(4))+u(2)*sin(u(4)-2*pi/3)+u(3)*sin(u(4)-4*pi/3))
  abc2q : Fcn  Expr=2/3*(u(1)*cos(u(4))+u(2)*cos(u(4)-2*pi/3)+u(3)*cos(u(4)-4*pi/3))
  dq : Outport  VectorParamsAs1DForOutWhenUnconnected=off
  wires:
  Mux2/1 -> dq/1
  abc2d/1 -> Mux2/2
  abc2q/1 -> Mux2/1
  Mux1/1 -> abc2d/1, abc2q/1
  theta/1 -> Mux1/2
  abc/1 -> Mux1/1

== system FOC_PMSM_FVSensorNew/PMSM motor/dq 2 afa beta ==
  dq : Inport
  theta : Inport  Port=2
  Mux1 : Mux  Inputs=2
  Mux2 : Mux  Inputs=2
  dq2afa : Fcn  Expr=u(1)*cos(u(3))-u(2)*sin(u(3))
  dq2beta : Fcn  Expr=u(1)*sin(u(3))+u(2)*cos(u(3))
  afa beta : Outport  VectorParamsAs1DForOutWhenUnconnected=off
  wires:
  dq/1 -> Mux1/1
  theta/1 -> Mux1/2
  Mux1/1 -> dq2beta/1, dq2afa/1
  dq2afa/1 -> Mux2/1
  dq2beta/1 -> Mux2/2
  Mux2/1 -> afa beta/1

== system FOC_PMSM_FVSensorNew/PMSM motor/dq0 2 abc ==
  dq0 : Inport
  theta : Inport  Port=2
  Mux1 : Mux  Inputs=2
  Mux2 : Mux  Inputs=3
  qd2a : Fcn  Expr=u(1)*cos(u(4))-u(2)*sin(u(4))+u(3)
  qd2b : Fcn  Expr=u(1)*cos(u(4)-2/3*pi)-u(2)*sin(u(4)-2/3*pi)+u(3)
  qd2c : Fcn  Expr=u(1)*cos(u(4)+2/3*pi)-u(2)*sin(u(4)+2/3*pi)+u(3)
  abc : Outport  VectorParamsAs1DForOutWhenUnconnected=off
  wires:
  Mux2/1 -> abc/1
  qd2b/1 -> Mux2/2
  qd2a/1 -> Mux2/1
  Mux1/1 -> qd2b/1, qd2c/1, qd2a/1
  theta/1 -> Mux1/2
  dq0/1 -> Mux1/1
  qd2c/1 -> Mux2/3

== system FOC_PMSM_FVSensorNew/PMSM motor/dq0 2 abc1 ==
  dq0 : Inport
  theta : Inport  Port=2
  Mux1 : Mux  Inputs=2
  Mux2 : Mux  Inputs=3
  qd2a : Fcn  Expr=u(1)*cos(u(4))-u(2)*sin(u(4))+u(3)
  qd2b : Fcn  Expr=u(1)*cos(u(4)-2/3*pi)-u(2)*sin(u(4)-2/3*pi)+u(3)
  qd2c : Fcn  Expr=u(1)*cos(u(4)+2/3*pi)-u(2)*sin(u(4)+2/3*pi)+u(3)
  abc : Outport  VectorParamsAs1DForOutWhenUnconnected=off
  wires:
  qd2c/1 -> Mux2/3
  dq0/1 -> Mux1/1
  theta/1 -> Mux1/2
  Mux1/1 -> qd2a/1, qd2c/1, qd2b/1
  qd2a/1 -> Mux2/1
  qd2b/1 -> Mux2/2
  Mux2/1 -> abc/1

== system FOC_PMSM_FVSensorNew/Pulse injection/afabet 2 abc ==
  afabet : Inport
  Constant : Constant  Value=0
  Mux1 : Mux  Inputs=2
  Mux2 : Mux  Inputs=3
  qd2a : Fcn  Expr=u(1)+u(3)
  qd2b : Fcn  Expr=u(1)*cos(2/3*pi)+u(2)*sin(2/3*pi)+u(3)
  qd2c : Fcn  Expr=u(1)*cos(2/3*pi)-u(2)*sin(2/3*pi)+u(3)
  abc : Outport  VectorParamsAs1DForOutWhenUnconnected=off
  wires:
  Constant/1 -> Mux1/2
  qd2c/1 -> Mux2/3
  afabet/1 -> Mux1/1
  Mux1/1 -> qd2c/1, qd2b/1, qd2a/1
  qd2a/1 -> Mux2/1
  qd2b/1 -> Mux2/2
  Mux2/1 -> abc/1

== system FOC_PMSM_FVSensorNew/Pulse injection/dq 2 afa beta ==
  dq : Inport
  theta : Inport  Port=2
  Mux1 : Mux  Inputs=2
  Mux2 : Mux  Inputs=2
  dq2afa : Fcn  Expr=u(1)*cos(u(3))-u(2)*sin(u(3))
  dq2beta : Fcn  Expr=u(1)*sin(u(3))+u(2)*cos(u(3))
  afa beta : Outport  VectorParamsAs1DForOutWhenUnconnected=off
  wires:
  dq/1 -> Mux1/1
  theta/1 -> Mux1/2
  Mux1/1 -> dq2beta/1, dq2afa/1
  dq2afa/1 -> Mux2/1
  dq2beta/1 -> Mux2/2
  Mux2/1 -> afa beta/1

== system FOC_PMSM_FVSensorNew/Rotor Pos. estimation/Cal. stator flux linkage ==
  v_in : Inport
  i_in : Inport  Port=2
  Discrete-Time Integrator : DiscreteIntegrator  SampleTime=-1  ICPrevOutput=DiscIntNeverNeededParam  ICPrevScaledInput=DiscIntNeverNeededParam
  Gain : Gain  Gain=Rs/2
  MinMax detection : Subsystem
  Scope6 : Scope
  Sum1 : Sum  Inputs=|+-
  Sum2 : Sum  Inputs=|+-
  Terminator : Terminator
  Terminator1 : Terminator
  Lndafa : Outport  VectorParamsAs1DForOutWhenUnconnected=off
  wires:
  MinMax detection/3(average) -> Sum2/2, Scope6/1
  Sum2/1 -> Lndafa/1
  MinMax detection/1(max.ou) -> Terminator/1
  MinMax detection/2(min.ou) -> Terminator1/1
  Gain/1 -> Sum1/2
  v_in/1 -> Sum1/1
  i_in/1 -> Gain/1
  Sum1/1 -> Discrete-Time Integrator/1
  Discrete-Time Integrator/1 -> Sum2/1, MinMax detection/1(In)

== system FOC_PMSM_FVSensorNew/Rotor Pos. estimation/Cal. stator flux linkage1 ==
  v_in : Inport
  i_in : Inport  Port=2
  Discrete-Time Integrator : DiscreteIntegrator  SampleTime=-1  ICPrevOutput=DiscIntNeverNeededParam  ICPrevScaledInput=DiscIntNeverNeededParam
  Gain : Gain  Gain=Rs/2
  MinMax detection : Subsystem
  Scope6 : Scope
  Sum1 : Sum  Inputs=|+-
  Sum2 : Sum  Inputs=|+-
  Terminator : Terminator
  Terminator1 : Terminator
  Lndafa : Outport  VectorParamsAs1DForOutWhenUnconnected=off
  wires:
  Discrete-Time Integrator/1 -> Sum2/1, MinMax detection/1(In)
  Sum1/1 -> Discrete-Time Integrator/1
  i_in/1 -> Gain/1
  v_in/1 -> Sum1/1
  Gain/1 -> Sum1/2
  MinMax detection/2(min.ou) -> Terminator1/1
  MinMax detection/1(max.ou) -> Terminator/1
  Sum2/1 -> Lndafa/1
  MinMax detection/3(average) -> Sum2/2, Scope6/1

== system FOC_PMSM_FVSensorNew/Vector Controller.discrete/Back EMF decoupling ==
  vdq,PI : Inport
  idq_meas : Inport  Port=2
  wr : Inport  Port=3
  Demux1 : Demux  Outputs=2
  Demux2 : Demux  Outputs=2
  Gain : Gain  Gain=Lq
  Gain1 : Gain  Gain=Ld
  Lndmpm : Constant  Value=Lndmpm
  Mux2 : Mux  Inputs=2
  Product : Product  RndMeth=Zero
  Product1 : Product  RndMeth=Zero
  Product2 : Product  RndMeth=Zero
  Sum : Sum  Inputs=|+-
  Sum1 : Sum  Inputs=|++
  Sum2 : Sum  Inputs=|++
  udq_cmd : Outport  VectorParamsAs1DForOutWhenUnconnected=off
  wires:
  Mux2/1 -> udq_cmd/1
  vdq,PI/1 -> Demux1/1
  Demux1/1 -> Sum/1
  Sum/1 -> Mux2/1
  Demux1/2 -> Sum1/1
  idq_meas/1 -> Demux2/1
  wr/1 -> Product/2, Product1/1, Product2/2
  Product1/1 -> Sum/2
  Gain/1 -> Product1/2
  Demux2/2 -> Gain/1
  Lndmpm/1 -> Product/1
  Product/1 -> Sum1/2
  Sum1/1 -> Sum2/1
  Demux2/1 -> Gain1/1
  Gain1/1 -> Product2/1
  Product2/1 -> Sum2/2
  Sum2/1 -> Mux2/2

== system FOC_PMSM_FVSensorNew/Vector Controller.discrete/PI controller.2 ==
  id_err : Inport
  Discrete-Time Integrator : DiscreteIntegrator  SampleTime=-1  ICPrevOutput=DiscIntNeverNeededParam  ICPrevScaledInput=DiscIntNeverNeededParam
  Kp : Gain  Gain=Kp2
  Sum1 : Sum  Inputs=|++
  ki : Gain  Gain=Ki2
  vd : Outport  VectorParamsAs1DForOutWhenUnconnected=off
  wires:
  Sum1/1 -> vd/1
  Discrete-Time Integrator/1 -> Sum1/2
  ki/1 -> Discrete-Time Integrator/1
  Kp/1 -> Sum1/1
  id_err/1 -> ki/1, Kp/1

== system FOC_PMSM_FVSensorNew/Vector Controller.discrete/PI controller.3 ==
  iq_err : Inport
  Discrete-Time Integrator : DiscreteIntegrator  SampleTime=-1  ICPrevOutput=DiscIntNeverNeededParam  ICPrevScaledInput=DiscIntNeverNeededParam
  Kp : Gain  Gain=8
  Sum1 : Sum  Inputs=|++
  ki : Gain  Gain=5000
  vq : Outport  VectorParamsAs1DForOutWhenUnconnected=off
  wires:
  Sum1/1 -> vq/1
  Discrete-Time Integrator/1 -> Sum1/2
  ki/1 -> Discrete-Time Integrator/1
  Kp/1 -> Sum1/1
  iq_err/1 -> ki/1, Kp/1

== system FOC_PMSM_FVSensorNew/Vector Controller.discrete/dq 2 afa beta ==
  dq : Inport
  theta : Inport  Port=2
  Mux1 : Mux  Inputs=2
  Mux2 : Mux  Inputs=2
  dq2afa : Fcn  Expr=u(1)*cos(u(3))-u(2)*sin(u(3))
  dq2beta : Fcn  Expr=u(1)*sin(u(3))+u(2)*cos(u(3))
  afa beta : Outport  VectorParamsAs1DForOutWhenUnconnected=off
  wires:
  Mux2/1 -> afa beta/1
  dq2beta/1 -> Mux2/2
  dq2afa/1 -> Mux2/1
  Mux1/1 -> dq2afa/1, dq2beta/1
  theta/1 -> Mux1/2
  dq/1 -> Mux1/1

== system FOC_PMSM_FVSensorNew/PLL/Scope/ InputMux  ==
  In1 : Inport
  Convert1 : DataTypeConversion  SaturateOnIntegerOverflow=on  RndMeth=Zero
  Mux : Mux  Inputs=1
  Out : Outport  VectorParamsAs1DForOutWhenUnconnected=off
  wires:
  Convert1/1 -> Mux/1
  In1/1 -> Convert1/1
  Mux/1 -> Out/1

== system FOC_PMSM_FVSensorNew/PMSM motor/Scope2/ InputMux  ==
  In1 : Inport
  Convert1 : DataTypeConversion  SaturateOnIntegerOverflow=on  RndMeth=Zero
  Mux : Mux  Inputs=1
  Out : Outport  VectorParamsAs1DForOutWhenUnconnected=off
  wires:
  Convert1/1 -> Mux/1
  In1/1 -> Convert1/1
  Mux/1 -> Out/1

== system FOC_PMSM_FVSensorNew/PMSM motor/Scope3/ InputMux  ==
  In1 : Inport
  Convert1 : DataTypeConversion  SaturateOnIntegerOverflow=on  RndMeth=Zero
  Mux : Mux  Inputs=1
  Out : Outport  VectorParamsAs1DForOutWhenUnconnected=off
  wires:
  Mux/1 -> Out/1
  In1/1 -> Convert1/1
  Convert1/1 -> Mux/1

== system FOC_PMSM_FVSensorNew/PMSM motor/Scope4/ InputMux  ==
  In1 : Inport
  Convert1 : DataTypeConversion  SaturateOnIntegerOverflow=on  RndMeth=Zero
  Mux : Mux  Inputs=1
  Out : Outport  VectorParamsAs1DForOutWhenUnconnected=off
  wires:
  Convert1/1 -> Mux/1
  In1/1 -> Convert1/1
  Mux/1 -> Out/1

== system FOC_PMSM_FVSensorNew/Rotor Pos. estimation/Cal. stator flux linkage/MinMax detection ==
  In : Inport
  Gain : Gain  Gain=1/2
  Max. Det : Subsystem
  Min. Det : Subsystem
  Mux6 : Mux  Inputs=3
  Scope5 : Scope
  Sum : Sum  Inputs=|++
  max.ou : Outport  VectorParamsAs1DForOutWhenUnconnected=off
  min.ou : Outport  Port=2  VectorParamsAs1DForOutWhenUnconnected=off
  average : Outport  Port=3  VectorParamsAs1DForOutWhenUnconnected=off
  wires:
  Gain/1 -> average/1
  Sum/1 -> Gain/1
  Max. Det/1(Max) -> max.ou/1, Mux6/1, Sum/1
  Min. Det/1(Min) -> min.ou/1, Mux6/3, Sum/2
  Mux6/1 -> Scope5/1
  In/1 -> Max. Det/1(In), Min. Det/1(In), Mux6/2

== system FOC_PMSM_FVSensorNew/Rotor Pos. estimation/Cal. stator flux linkage1/MinMax detection ==
  In : Inport
  Gain : Gain  Gain=1/2
  Max. Det : Subsystem
  Min. Det : Subsystem
  Mux6 : Mux  Inputs=3
  Scope5 : Scope
  Sum : Sum  Inputs=|++
  max.ou : Outport  VectorParamsAs1DForOutWhenUnconnected=off
  min.ou : Outport  Port=2  VectorParamsAs1DForOutWhenUnconnected=off
  average : Outport  Port=3  VectorParamsAs1DForOutWhenUnconnected=off
  wires:
  Gain/1 -> average/1
  Sum/1 -> Gain/1
  Max. Det/1(Max) -> max.ou/1, Mux6/1, Sum/1
  Min. Det/1(Min) -> min.ou/1, Mux6/3, Sum/2
  Mux6/1 -> Scope5/1
  In/1 -> Max. Det/1(In), Min. Det/1(In), Mux6/2

== system FOC_PMSM_FVSensorNew/Rotor Pos. estimation/Cal. stator flux linkage/MinMax detection/Max. Det ==
  In : Inport
  Counter.1 : Subsystem
  Counter.2 : Subsystem
  Gain1 : Gain
  Gain2 : Gain  Gain=0.3
  Gain3 : Gain  Gain=0.6
  Mux2 : Mux
  Product : Product  RndMeth=Zero
  Relational Operator : RelationalOperator  RndMeth=Nearest
  Scope3 : Scope
  Unit Delay : UnitDelay  SampleTime=-1  HasFrameUpgradeWarning=on
  max.1 : Subsystem
  max.3 : Subsystem
  Max : Outport  VectorParamsAs1DForOutWhenUnconnected=off
  wires:
  Unit Delay/1 -> Relational Operator/2
  In/1 -> Unit Delay/1, max.1/1(In), Relational Operator/1, Mux2/1
  Relational Operator/1 -> max.1/Trigger, Counter.1/1(Sig.In), Counter.2/1(Sig.In), Gain1/1
  max.1/1(Out) -> max.3/1(In)
  Counter.1/1(En) -> Product/2, Gain3/1
  Mux2/1 -> Scope3/1
  Counter.2/1(En) -> Product/1, Gain2/1
  Product/1 -> max.3/Trigger
  Gain1/1 -> Mux2/2
  Gain2/1 -> Mux2/3
  Gain3/1 -> Mux2/4
  max.3/1(Out) -> Max/1

== system FOC_PMSM_FVSensorNew/Rotor Pos. estimation/Cal. stator flux linkage/MinMax detection/Min. Det ==
  In : Inport
  Counter.1 : Subsystem
  Counter.2 : Subsystem
  Gain1 : Gain
  Gain2 : Gain  Gain=0.3
  Gain3 : Gain  Gain=0.6
  Mux2 : Mux
  Product : Product  RndMeth=Zero
  Relational Operator : RelationalOperator  Operator=<=  RndMeth=Nearest
  Scope3 : Scope
  Unit Delay : UnitDelay  SampleTime=-1  HasFrameUpgradeWarning=on
  max.1 : Subsystem
  max.3 : Subsystem
  Min : Outport  VectorParamsAs1DForOutWhenUnconnected=off
  wires:
  max.3/1(Out) -> Min/1
  Gain3/1 -> Mux2/4
  Gain2/1 -> Mux2/3
  Gain1/1 -> Mux2/2
  Product/1 -> max.3/Trigger
  Counter.2/1(En) -> Gain2/1, Product/1
  Mux2/1 -> Scope3/1
  Counter.1/1(En) -> Gain3/1, Product/2
  max.1/1(Out) -> max.3/1(In)
  Relational Operator/1 -> Gain1/1, Counter.2/1(Sig.In), Counter.1/1(Sig.In), max.1/Trigger
  In/1 -> Mux2/1, Relational Operator/1, max.1/1(In), Unit Delay/1
  Unit Delay/1 -> Relational Operator/2

== system FOC_PMSM_FVSensorNew/Rotor Pos. estimation/Cal. stator flux linkage1/MinMax detection/Max. Det ==
  In : Inport
  Counter.1 : Subsystem
  Counter.2 : Subsystem
  Gain1 : Gain
  Gain2 : Gain  Gain=0.3
  Gain3 : Gain  Gain=0.6
  Mux2 : Mux
  Product : Product  RndMeth=Zero
  Relational Operator : RelationalOperator  RndMeth=Nearest
  Scope3 : Scope
  Unit Delay : UnitDelay  SampleTime=-1  HasFrameUpgradeWarning=on
  max.1 : Subsystem
  max.3 : Subsystem
  Max : Outport  VectorParamsAs1DForOutWhenUnconnected=off
  wires:
  Unit Delay/1 -> Relational Operator/2
  In/1 -> Unit Delay/1, max.1/1(In), Relational Operator/1, Mux2/1
  Relational Operator/1 -> max.1/Trigger, Counter.1/1(Sig.In), Counter.2/1(Sig.In), Gain1/1
  max.1/1(Out) -> max.3/1(In)
  Counter.1/1(En) -> Product/2, Gain3/1
  Mux2/1 -> Scope3/1
  Counter.2/1(En) -> Product/1, Gain2/1
  Product/1 -> max.3/Trigger
  Gain1/1 -> Mux2/2
  Gain2/1 -> Mux2/3
  Gain3/1 -> Mux2/4
  max.3/1(Out) -> Max/1

== system FOC_PMSM_FVSensorNew/Rotor Pos. estimation/Cal. stator flux linkage1/MinMax detection/Min. Det ==
  In : Inport
  Counter.1 : Subsystem
  Counter.2 : Subsystem
  Gain1 : Gain
  Gain2 : Gain  Gain=0.3
  Gain3 : Gain  Gain=0.6
  Mux2 : Mux
  Product : Product  RndMeth=Zero
  Relational Operator : RelationalOperator  Operator=<=  RndMeth=Nearest
  Scope3 : Scope
  Unit Delay : UnitDelay  SampleTime=-1  HasFrameUpgradeWarning=on
  max.1 : Subsystem
  max.3 : Subsystem
  Min : Outport  VectorParamsAs1DForOutWhenUnconnected=off
  wires:
  max.3/1(Out) -> Min/1
  Gain3/1 -> Mux2/4
  Gain2/1 -> Mux2/3
  Gain1/1 -> Mux2/2
  Product/1 -> max.3/Trigger
  Counter.2/1(En) -> Gain2/1, Product/1
  Mux2/1 -> Scope3/1
  Counter.1/1(En) -> Gain3/1, Product/2
  max.1/1(Out) -> max.3/1(In)
  Relational Operator/1 -> Gain1/1, Counter.2/1(Sig.In), Counter.1/1(Sig.In), max.1/Trigger
  In/1 -> Mux2/1, Relational Operator/1, max.1/1(In), Unit Delay/1
  Unit Delay/1 -> Relational Operator/2

== system FOC_PMSM_FVSensorNew/Rotor Pos. estimation/Cal. stator flux linkage/MinMax detection/Max. Det/Counter.1 ==
  Sig.In : Inport
  Constant4 : Constant  Value=10
  Constant5 : Constant
  Conter with enable : Subsystem
  Sum1 : Sum  Inputs=|-+
  En : Outport  VectorParamsAs1DForOutWhenUnconnected=off
  wires:
  Constant5/1 -> Sum1/2
  Sig.In/1 -> Sum1/1
  Conter with enable/1(Max. Reached?) -> En/1
  Sum1/1 -> Conter with enable/1(_|  |_)
  Constant4/1 -> Conter with enable/2(Max. Num)

== system FOC_PMSM_FVSensorNew/Rotor Pos. estimation/Cal. stator flux linkage/MinMax detection/Max. Det/Counter.2 ==
  Sig.In : Inport
  Constant4 : Constant  Value=5
  Conter with enable : Subsystem
  Gain : Gain  Gain=2
  Gain1 : Gain  Gain=3
  Gain2 : Gain  Gain=4
  Mux1 : Mux
  Rising edge gen. : Subsystem
  SR Latch : Subsystem
  Scope2 : Scope
  En : Outport  VectorParamsAs1DForOutWhenUnconnected=off
  wires:
  Constant4/1 -> Conter with enable/2(Max. Num)
  Sig.In/1 -> Conter with enable/1(_|  |_), Rising edge gen./1(_|  |_), Gain2/1
  Conter with enable/1(Max. Reached?) -> SR Latch/2(S), Gain1/1
  SR Latch/1(Q) -> En/1, Mux1/1
  Mux1/1 -> Scope2/1
  Rising edge gen./1(Edge) -> SR Latch/1(R), Gain/1
  Gain/1 -> Mux1/2
  Gain1/1 -> Mux1/3
  Gain2/1 -> Mux1/4

== system FOC_PMSM_FVSensorNew/Rotor Pos. estimation/Cal. stator flux linkage/MinMax detection/Max. Det/max.1 ==
  In : Inport
  Trigger : TriggerPort  TriggerType=falling  VariantControl=(inherit)
  Out : Outport  VectorParamsAs1DForOutWhenUnconnected=off
  wires:
  In/1 -> Out/1

== system FOC_PMSM_FVSensorNew/Rotor Pos. estimation/Cal. stator flux linkage/MinMax detection/Max. Det/max.3 ==
  In : Inport
  Trigger : TriggerPort  VariantControl=(inherit)
  Out : Outport  VectorParamsAs1DForOutWhenUnconnected=off
  wires:
  In/1 -> Out/1

== system FOC_PMSM_FVSensorNew/Rotor Pos. estimation/Cal. stator flux linkage/MinMax detection/Min. Det/Counter.1 ==
  Sig.In : Inport
  Constant4 : Constant  Value=10
  Constant5 : Constant
  Conter with enable : Subsystem
  Sum1 : Sum  Inputs=|-+
  En : Outport  VectorParamsAs1DForOutWhenUnconnected=off
  wires:
  Constant4/1 -> Conter with enable/2(Max. Num)
  Sum1/1 -> Conter with enable/1(_|  |_)
  Conter with enable/1(Max. Reached?) -> En/1
  Sig.In/1 -> Sum1/1
  Constant5/1 -> Sum1/2

== system FOC_PMSM_FVSensorNew/Rotor Pos. estimation/Cal. stator flux linkage/MinMax detection/Min. Det/Counter.2 ==
  Sig.In : Inport
  Constant4 : Constant  Value=5
  Conter with enable : Subsystem
  Gain : Gain  Gain=2
  Gain1 : Gain  Gain=3
  Gain2 : Gain  Gain=4
  Mux1 : Mux
  Rising edge gen. : Subsystem
  SR Latch : Subsystem
  Scope2 : Scope
  En : Outport  VectorParamsAs1DForOutWhenUnconnected=off
  wires:
  Gain2/1 -> Mux1/4
  Gain1/1 -> Mux1/3
  Gain/1 -> Mux1/2
  Rising edge gen./1(Edge) -> Gain/1, SR Latch/1(R)
  Mux1/1 -> Scope2/1
  SR Latch/1(Q) -> Mux1/1, En/1
  Conter with enable/1(Max. Reached?) -> Gain1/1, SR Latch/2(S)
  Sig.In/1 -> Gain2/1, Rising edge gen./1(_|  |_), Conter with enable/1(_|  |_)
  Constant4/1 -> Conter with enable/2(Max. Num)

== system FOC_PMSM_FVSensorNew/Rotor Pos. estimation/Cal. stator flux linkage/MinMax detection/Min. Det/max.1 ==
  In : Inport
  Trigger : TriggerPort  TriggerType=falling  VariantControl=(inherit)
  Out : Outport  VectorParamsAs1DForOutWhenUnconnected=off
  wires:
  In/1 -> Out/1

== system FOC_PMSM_FVSensorNew/Rotor Pos. estimation/Cal. stator flux linkage/MinMax detection/Min. Det/max.3 ==
  In : Inport
  Trigger : TriggerPort  VariantControl=(inherit)
  Out : Outport  VectorParamsAs1DForOutWhenUnconnected=off
  wires:
  In/1 -> Out/1

== system FOC_PMSM_FVSensorNew/Rotor Pos. estimation/Cal. stator flux linkage1/MinMax detection/Max. Det/Counter.1 ==
  Sig.In : Inport
  Constant4 : Constant  Value=10
  Constant5 : Constant
  Conter with enable : Subsystem
  Sum1 : Sum  Inputs=|-+
  En : Outport  VectorParamsAs1DForOutWhenUnconnected=off
  wires:
  Constant5/1 -> Sum1/2
  Sig.In/1 -> Sum1/1
  Conter with enable/1(Max. Reached?) -> En/1
  Sum1/1 -> Conter with enable/1(_|  |_)
  Constant4/1 -> Conter with enable/2(Max. Num)

== system FOC_PMSM_FVSensorNew/Rotor Pos. estimation/Cal. stator flux linkage1/MinMax detection/Max. Det/Counter.2 ==
  Sig.In : Inport
  Constant4 : Constant  Value=5
  Conter with enable : Subsystem
  Gain : Gain  Gain=2
  Gain1 : Gain  Gain=3
  Gain2 : Gain  Gain=4
  Mux1 : Mux
  Rising edge gen. : Subsystem
  SR Latch : Subsystem
  Scope2 : Scope
  En : Outport  VectorParamsAs1DForOutWhenUnconnected=off
  wires:
  Constant4/1 -> Conter with enable/2(Max. Num)
  Sig.In/1 -> Conter with enable/1(_|  |_), Rising edge gen./1(_|  |_), Gain2/1
  Conter with enable/1(Max. Reached?) -> SR Latch/2(S), Gain1/1
  SR Latch/1(Q) -> En/1, Mux1/1
  Mux1/1 -> Scope2/1
  Rising edge gen./1(Edge) -> SR Latch/1(R), Gain/1
  Gain/1 -> Mux1/2
  Gain1/1 -> Mux1/3
  Gain2/1 -> Mux1/4

== system FOC_PMSM_FVSensorNew/Rotor Pos. estimation/Cal. stator flux linkage1/MinMax detection/Max. Det/max.1 ==
  In : Inport
  Trigger : TriggerPort  TriggerType=falling  VariantControl=(inherit)
  Out : Outport  VectorParamsAs1DForOutWhenUnconnected=off
  wires:
  In/1 -> Out/1

== system FOC_PMSM_FVSensorNew/Rotor Pos. estimation/Cal. stator flux linkage1/MinMax detection/Max. Det/max.3 ==
  In : Inport
  Trigger : TriggerPort  VariantControl=(inherit)
  Out : Outport  VectorParamsAs1DForOutWhenUnconnected=off
  wires:
  In/1 -> Out/1

== system FOC_PMSM_FVSensorNew/Rotor Pos. estimation/Cal. stator flux linkage1/MinMax detection/Min. Det/Counter.1 ==
  Sig.In : Inport
  Constant4 : Constant  Value=10
  Constant5 : Constant
  Conter with enable : Subsystem
  Sum1 : Sum  Inputs=|-+
  En : Outport  VectorParamsAs1DForOutWhenUnconnected=off
  wires:
  Constant4/1 -> Conter with enable/2(Max. Num)
  Sum1/1 -> Conter with enable/1(_|  |_)
  Conter with enable/1(Max. Reached?) -> En/1
  Sig.In/1 -> Sum1/1
  Constant5/1 -> Sum1/2
